simulink model "controller_template_vTST"  (Simulink 7.8)
settings: Solver=ode45  SolverMode=SingleTasking  StartTime=0.0  StopTime=20  FixedStep=Ts  RelTol=1e-3
PreLoadFcn:
  | load_waypoints
values from neighbouring files (symbols this model uses):
  Aff_pitch = [0.764669359834 -6.55628329998 -0.0099932514458 -0.411590904828 0.0133529191446 -0.0326334422872 -8.8646944178e-05 -0.00470014240893 0 0 1 0 ... (16 elements, 4x4)]    [kostas_malakies.mat]    (also in kostas_malakies2.mat)
  Aff_roll = [0.825180563081 -6.10606264808 -0.00763580464276 -0.367448917026 0.0145694646817 0.0253169520582 -6.457583527e-05 -0.00409059128644 0 0 1 0 ... (16 elements, 4x4)]    [kostas_malakies.mat]    (also in kostas_malakies2.mat; main_last.m = [Aff_roll,zeros(size(Aff_roll,1),1);zeros(1,size(Aff_roll,1))
  Aff_yaw = 0.520554464036    [kostas_malakies.mat]    (also in kostas_malakies2.mat; main.m = sysfd_yaw.a; main_last.m = sysfd_yaw.a)
  Bff_pitch = [0.235330640166  0; 6.55628329998  0; -0.000567656018985  0; -0.0435256495914  0]    [kostas_malakies.mat]    (also in kostas_malakies2.mat)
  Bff_roll = [0.174819436919  0; 6.10606264808  0; -0.000299760068643  0; -0.0270637325616  0]    [kostas_malakies.mat]    (also in kostas_malakies2.mat; main_last.m = [Bff_roll;zeros(1,size(Bff_roll,2))])
  Bff_yaw = 0.479445535964    [kostas_malakies.mat]    (also in kostas_malakies2.mat; main.m = sysfd_yaw.b; main_last.m = sysfd_yaw.b)
  Fi_XdirFF = [-0.447351940284 0 0 -1.28434394361 -4.04417159595 -1.80654990505 -1.28434394361 1 -4.04417159595 -1.80654990505 1 0 ... (536 elements, 134x4)]    [kostas_malakies.mat]    (also in kostas_malakies2.mat; matlab.mat = [-1.62441280603 -1.28434394361 -1.7723315065 -1.66810627541 )
  Fi_Yaw = [-1.14619813144 0 0]    [kostas_malakies.mat]    (also in kostas_malakies2.mat; matlab.mat = -0.284754025426)
  Fi_Ydir = [-0.466308586531 2.22044604925e-16 2.22044604925e-16 -1.46518332723 -4.54395337171 -2.00318743375 -1.46518332723 1 -4.54395337171 -2.00318743375 1 2.22044604925e-16 ... (536 elements, 134x4)]    [kostas_malakies.mat]    (also in kostas_malakies2.mat = [-0.521298425559 -2.64128186917 -15.6565978667 -8.2066553194; matlab.mat = [1 -1.9173235349 -1.46518332723 1 1 1 1 1 -1.98764774833 -1.)
  Fi_Zdir = [0 -1.80359099426e-16 0 1.4149586889 0 0 2.30859647265e-14 -5.77149118162e-15 0 0 0 0 ... (54 elements, 27x2)]    [kostas_malakies.mat]    (also in kostas_malakies2.mat = [4.30976351396 0 4.73307471514 3.80948040666 0 0 0 0.5468933; matlab.mat = [0 -9.51943523339e-14 0 1.99761158231 0 1.18992940417e-14 0 )
  g = 9.8065    [kostas_malakies.mat]    (also in kostas_malakies2.mat; load_PMModel.m = 9.81; main.m; main_last.m)
  Gi_XdirFF = [0 0.27 -0.27 0.478341621792 -6.42962779272 -1.98615606962 -0.478341621792 -0.373552567526 6.42962779272 1.98615606962 0.373552567526 0.27 ... (134 elements, 134x1)]    [kostas_malakies.mat]    (also in kostas_malakies2.mat; matlab.mat = [3.88578058619e-16 0.478341621792 -0.139455879222 -0.1159311)
  Gi_Yaw = [4.4408920985e-16 -3.14159265359 3.14159265359]    [kostas_malakies.mat]    (also in kostas_malakies2.mat = [-4.4408920985e-16 -3.14159265359 3.14159265359]; matlab.mat = 4.4408920985e-16)
  Gi_Ydir = [-2.77555756156e-16 0.27 -0.27 0.516209388722 7.06668201156 2.10835273651 -0.516209388722 -0.383863816771 -7.06668201156 -2.10835273651 0.383863816771 0.27 ... (134 elements, 134x1)]    [kostas_malakies.mat]    (also in kostas_malakies2.mat = [1.11022302463e-16 0.765579126644 531.260413192 11.754237275; matlab.mat = [0.383863816771 -0.133207088705 0.516209388722 0.38386381677)
  Gi_Zdir = [-1 -1 -1 2.22044604925e-16 -1 -1 -1 -1 1 -1 -1 -1 ... (27 elements, 27x1)]    [kostas_malakies.mat]    (also in kostas_malakies2.mat = [0.174387892495 -1 0.368373831608 3.33066907388e-16 -1 -1 -1; matlab.mat = [-2 -2 -2 1.11022302463e-15 -2 -2 -2 2 -2 -2 -2 2 ... (21 el)
  Hn_XdirFF = [-0.618529611748 0.618529611748 0.827215259158 -0.512155371354 -0.650909395739 -0.827215259158 0.930717154057 0.512155371354 0.650909395739 -0.930717154057 -1 0 ... (4464 elements, 1116x4)]    [kostas_malakies.mat]    (also in kostas_malakies2.mat; matlab.mat = [1 -0.136019433325 -0.405248495598 -0.339279056031 0 -1 0.13)
  Hn_Yaw = [1 -1 -1 1 1 -1]    [kostas_malakies.mat]    (also in kostas_malakies2.mat; matlab.mat = [1 -1])
  Hn_Ydir = [-0.642151612842 0.642151612842 0.873369621238 0.521434628645 0.668917219747 -0.873369621238 0.934789012395 -0.521434628645 -0.668917219747 -0.934789012395 -1 0 ... (4532 elements, 1133x4)]    [kostas_malakies.mat]    (also in kostas_malakies2.mat = [0.972602710123 0.0284063109089 0.559530157965 0.73050130567; matlab.mat = [0.711566553558 0.999813894311 -0.735660470031 0 0 0.5471922)
  Hn_Zdir = [-0.560552458797 -0.996815278536 -0.988320507921 0.666673243042 -1 0 -0.421994354267 -0.987440631917 -0.973284290019 -0.956170964903 -0.936236606521 0.560552458797 ... (224 elements, 112x2)]    [kostas_malakies.mat]    (also in kostas_malakies2.mat = [-0.781813705838 -0.712499731132 0.751798766698 0 -0.7286973; matlab.mat = [1 -1 -0.996815278536 -0.990718937584 -0.276007160242 0.3840)
  Kn_XdirFF = [0.373314565409 0.373314565409 0.472754204418 0.915522246067 0.951154784392 0.472754204418 0.240212330437 0.915522246067 0.951154784392 0.240212330437 0.2094 2 ... (1116 elements, 1116x1)]    [kostas_malakies.mat]    (also in kostas_malakies2.mat; matlab.mat = [0.2094 0.19132523886 0.382063154155 0.900203176458 2 0.2094)
  Kn_Yaw = [2.74088097634 2.74088097634 -2.74088097634 3.14159265359 -2.74088097634 3.14159265359]    [kostas_malakies.mat]    (also in kostas_malakies2.mat; matlab.mat = [0.0873 0.0873])
  Kn_Ydir = [0.371815875743 0.371815875743 0.451349483511 0.90366201682 0.917647772499 0.451349483511 0.24471770913 0.90366201682 0.917647772499 0.24471770913 0.2094 2 ... (1133 elements, 1133x1)]    [kostas_malakies.mat]    (also in kostas_malakies2.mat = [0.351231202126 0.997082913977 0.855763802521 0.792250278627; matlab.mat = [-0.126119149197 0.0536759032179 0.37354703421 2 2 -0.239682)
  Kn_Zdir = [0.727672356179 1.00172267683 1.00656919451 -0.471160923828 1 1 1.18526984431 1.00688561667 1.01272393898 1.01603878926 1.01572683497 -0.727672356179 ... (112 elements, 112x1)]    [kostas_malakies.mat]    (also in kostas_malakies2.mat = [0.21304012328 0.326509029469 -0.262060822346 1 0.301409884 ; matlab.mat = [1 1 1.00663007512 1.02122194908 0.632590992205 -0.384463644)
  Nc_XdirFF = [18 15 15 11 9 7 11 14 9 7 14 8 ... (134 elements, 134x1)]    [kostas_malakies.mat]    (also in kostas_malakies2.mat; matlab.mat = [14 8 7 10 8 7 10 12 10 10 12 11 ... (107 elements, 107x1)])
  Nc_Yaw = [2 2 2]    [kostas_malakies.mat]    (also in kostas_malakies2.mat; matlab.mat = 2)
  Nc_Ydir = [18 16 16 10 9 7 10 14 9 7 14 8 ... (134 elements, 134x1)]    [kostas_malakies.mat]    (also in kostas_malakies2.mat = [22 12 6 9 9 5 12 13 6 9 9 5 ... (171 elements, 171x1)]; matlab.mat = [11 8 12 15 7 9 10 13 10 14 12 7 ... (104 elements, 104x1)])
  Nc_Zdir = [6 7 3 6 3 4 4 3 6 5 3 4 ... (27 elements, 27x1)]    [kostas_malakies.mat]    (also in kostas_malakies2.mat = [4 4 3 12 5 4 3 3 4 3 3 4 ... (93 elements, 93x1)]; matlab.mat = [6 3 7 4 4 3 4 6 3 5 3 3 ... (21 elements, 21x1)])
  pitch_cmd2pitch_1stOrd = 1.42468924998    [kostas_malakies.mat]    (also in kostas_malakies2.mat)
  roll_cmd2roll_1stOrd = 1.38101661575    [kostas_malakies.mat]    (also in kostas_malakies2.mat)
  thrust_cmd2thrust_0thOrd = 0.876575459522    [kostas_malakies.mat]    (also in kostas_malakies2.mat)
  THRUST_CMD_GAIN = -0.0835    [kostas_malakies.mat]    (also in kostas_malakies2.mat; load_PMModel.m)
  Ts = 0.02    [kostas_malakies.mat]    (also in kostas_malakies2.mat; main.m; main_last.m; matlab.mat = 0.08)
  yaw_cmd2yaw_1stOrd = 2.01792090263    [kostas_malakies.mat]    (also in kostas_malakies2.mat)
  z = [-0.93079906702 -0.933865725994 -0.937557637691 -0.939011216164 -0.94143640995 -0.944628417492 -0.947235524654 -0.949601888657 -0.952827751637 -0.9567258358 -0.958320975304 -0.960991024971 ... (7988 elements, 7988x1)]    [kostas_malakies2.mat]    (also in plotDataTest.m = simout_data.signals.values(:,11))
libraries: simulink x6, Hquad_control_LIB_MPC x5
(part 2 of 2)

== matlab function FreeFlight Pos Ctrl/MAIN CONTROL LOOP1/y controller MPC FG/Explicit Ctrl1/Ctrl_Xdir ==
  data: X input double; U output double; Hn input double; Kn input double; Fi input double; Gi input double; Nc input double; flag_oob output double
function [U,flag_oob] = OptimalMPCInput(X,Hn,Kn,Fi,Gi,Nc)

tolerance = 1;
nr  = size(Nc,1);
MPT_ABSTOL = 1e-8;
minreg = 0;
X = round(10000*X)/10000;

flag_oob = 0;
%maxSize = max(Nc);

Hi = zeros(100,4);
Ki = zeros(100,1);

% Find the proper region
abspos = 1;
for ireg = 1:nr
    sumViol = 0;
    isinside = 1;
    

  %  Hi(1:Nc(ireg),1:4) = Hn(abspos:(abspos+Nc(ireg)-1),1:4);
    for i = 1:Nc(ireg)
        for j = 1:4
            Hi(i,j) = Hn(abspos + i - 1,j);
        end
    end
    
%    Ki(1:Nc(ireg),1) = Kn(abspos:(abspos+Nc(ireg)-1),1);
    for i = 1:Nc(ireg)
        Ki(i,1) = Kn(abspos + i - 1,1);
    end
    abspos = abspos + Nc(ireg);
    
    F = Fi(ireg,:);
    G = Gi(ireg,:);
    
    nc = Nc(ireg);
    
    for ic = 1:nc
        hx = Hi(ic,:)*X;
        if ((hx - Ki(ic)) > MPT_ABSTOL)
            isinside = 0;
            sumViol = sumViol + (hx - Ki(ic));
        end
    end
    
    if (sumViol < tolerance)
        tolerance = sumViol;
        minreg = ireg;
    end
    % extract the right control law
    if (isinside == 1)
        U = F*X + G;
        return
    end
end
F = Fi(minreg,:);
G = Gi(minreg,:);
U = F*X + G;
flag_oob = 1;
%U = U_prev;
return

== matlab function FreeFlight Pos Ctrl/MAIN CONTROL LOOP1/z controller MPC FG/Explicit Ctrl1/Ctrl_Xdir ==
  data: X input double; U output double; Hn input double; Kn input double; Fi input double; Gi input double; Nc input double; flag_oob output double
function [U,flag_oob] = OptimalMPCInput(X,Hn,Kn,Fi,Gi,Nc)

tolerance = 1;
nr  = size(Nc,1);
MPT_ABSTOL = 1e-8;
minreg = 0;
X = round(10000*X)/10000;

flag_oob = 0;
%maxSize = max(Nc);

Hi = zeros(100,2);
Ki = zeros(100,1);

% Find the proper region
abspos = 1;
for ireg = 1:nr
    sumViol = 0;
    isinside = 1;
    

  %  Hi(1:Nc(ireg),1:4) = Hn(abspos:(abspos+Nc(ireg)-1),1:4);
    for i = 1:Nc(ireg)
        for j = 1:2
            Hi(i,j) = Hn(abspos + i - 1,j);
        end
    end
    
%    Ki(1:Nc(ireg),1) = Kn(abspos:(abspos+Nc(ireg)-1),1);
    for i = 1:Nc(ireg)
        Ki(i,1) = Kn(abspos + i - 1,1);
    end
    abspos = abspos + Nc(ireg);
    
    F = Fi(ireg,:);
    G = Gi(ireg,:);
    
    nc = Nc(ireg);
    
    for ic = 1:nc
        hx = Hi(ic,:)*X;
        if ((hx - Ki(ic)) > MPT_ABSTOL)
            isinside = 0;
            sumViol = sumViol + (hx - Ki(ic));
        end
    end
    
    if (sumViol < tolerance)
        tolerance = sumViol;
        minreg = ireg;
    end
    % extract the right control law
    if (isinside == 1)
        U = F*X + G;
        return
    end
end
F = Fi(minreg,:);
G = Gi(minreg,:);
U = F*X + G;
flag_oob = 1;
%U = U_prev;
return

== matlab function FreeFlight Pos Ctrl/MAIN CONTROL LOOP1/yaw controller MPC FG/Explicit Ctrl1/Ctrl_Xdir ==
  data: X input double; U output double; Hn input double; Kn input double; Fi input double; Gi input double; Nc input double; flag_oob output double
function [U,flag_oob] = OptimalMPCInput(X,Hn,Kn,Fi,Gi,Nc)

tolerance = 1;
nr  = size(Nc,1);
MPT_ABSTOL = 1e-8;
minreg = 0;
X = round(10000*X)/10000;

flag_oob = 0;
%maxSize = max(Nc);

Hi = zeros(100,1);
Ki = zeros(100,1);

% Find the proper region
abspos = 1;
for ireg = 1:nr
    sumViol = 0;
    isinside = 1;
    

  %  Hi(1:Nc(ireg),1:4) = Hn(abspos:(abspos+Nc(ireg)-1),1:4);
    for i = 1:Nc(ireg)
        for j = 1:1
            Hi(i,j) = Hn(abspos + i - 1,j);
        end
    end
    
%    Ki(1:Nc(ireg),1) = Kn(abspos:(abspos+Nc(ireg)-1),1);
    for i = 1:Nc(ireg)
        Ki(i,1) = Kn(abspos + i - 1,1);
    end
    abspos = abspos + Nc(ireg);
    
    F = Fi(ireg,:);
    G = Gi(ireg,:);
    
    nc = Nc(ireg);
    
    for ic = 1:nc
        hx = Hi(ic,:)*X;
        if ((hx - Ki(ic)) > MPT_ABSTOL)
            isinside = 0;
            sumViol = sumViol + (hx - Ki(ic));
        end
    end
    
    if (sumViol < tolerance)
        tolerance = sumViol;
        minreg = ireg;
    end
    % extract the right control law
    if (isinside == 1)
        U = F*X + G;
        return
    end
end
F = Fi(minreg,:);
G = Gi(minreg,:);
U = F*X + G;
flag_oob = 1;
%U = U_prev;
return

== matlab function FreeFlight Pos Ctrl/MAIN CONTROL LOOP1/y controller MPC FG/Explicit Ctrl1/RollPropagate/MATLAB Function ==
  data: x input double; y output double; A input double; B input double; u input double
function y = fcn(x,A,B,u)
%#codegen

y = A*x + B*[u;0];

== matlab function FreeFlight Pos Ctrl/MAIN CONTROL LOOP1/yaw controller MPC FG/Explicit Ctrl1/YawPropagate/MATLAB Function ==
  data: x input double; y output double; A input double; B input double; u input double
function y = fcn(x,A,B,u)
%#codegen

y = A*x + B*u;

== matlab function FreeFlight Pos Ctrl/MAIN CONTROL LOOP1/x controller MPC FG /Explicit Ctrl1/PitchPropagate/MATLAB Function ==
  data: x input double; y output double; A input double; B input double; u input double
function y = fcn(x,A,B,u)
%#codegen

y = A*x + B*[u;0];
